simulink model "gs"  (Simulink 8.5)
settings: Solver=ode8  StartTime=0.0  StopTime=200  FixedStep=0.1  RelTol=1e-3
settings Model: Creator=Default  LastModifiedBy=Default
settings DataIOCC: SignalLoggingSaveFormat=Dataset
settings OptimizationCC: ExpressionDepthLimit=128
settings DebuggingCC: UnderspecifiedInitializationDetection=Simplified  MergeDetectMultiDrivingBlocksExec=error  FcnCallInpInsideContextMsg=EnableAllAsError  StateNameClashWarn=none
settings GRTTargetCC: CombineOutputUpdateFcns=on  GRTInterface=off

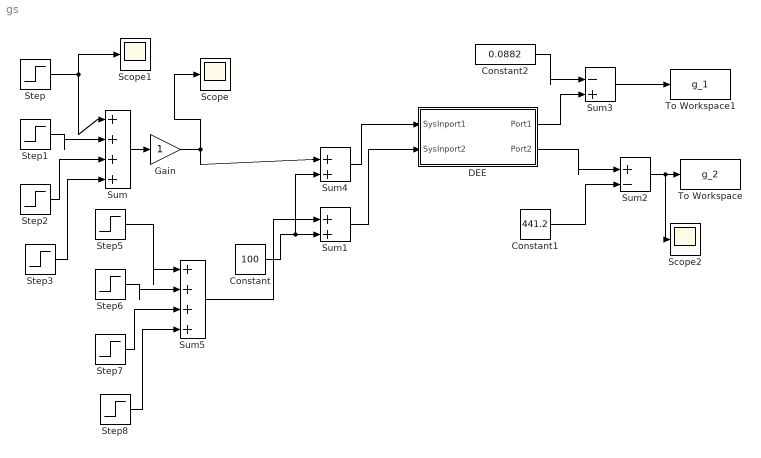
== system gs ==
  Constant : Constant  Value=100
  Constant1 : Constant  Value=441.2
  Constant2 : Constant  Value=0.0882
  DEE : Subsystem  mask(Differential Equation Editor (DEE)){}
      settings: OpenFcn=diffeqed
      mask Display: disp('Differential Equation\n Editor')
  Gain : Gain
  Scope : Scope
  Scope1 : Scope
  Scope2 : Scope
      settings: SaveName=ScopeData2
  Step : Step  Time=20  SampleTime=0
  Step1 : Step  Time=40  After=-1  SampleTime=0
  Step2 : Step  Time=60  After=-1  SampleTime=0
  Step3 : Step  Time=80  SampleTime=0
  Step5 : Step  Time=120  SampleTime=0
  Step6 : Step  Time=140  After=-1  SampleTime=0
  Step7 : Step  Time=160  After=-1  SampleTime=0
  Step8 : Step  Time=180  SampleTime=0
  Sum : Sum  Inputs=|++++
  Sum1 : Sum  Inputs=|++
  Sum2 : Sum  Inputs=|+-
  Sum3 : Sum  Inputs=|-+
  Sum4 : Sum  Inputs=|++
  Sum5 : Sum  Inputs=|++++
  To Workspace : ToWorkspace  VariableName=g_2  SampleTime=-1
  To Workspace1 : ToWorkspace  VariableName=g_1  SampleTime=-1
  wires:
  Step/1 -> Sum/1, Scope1/1
  Step1/1 -> Sum/2
  Step2/1 -> Sum/3
  Step3/1 -> Sum/4
  Sum/1 -> Gain/1
  Constant/1 -> Sum4/2, Sum1/2
  Constant1/1 -> Sum2/2
  Sum2/1 -> Scope2/1, To Workspace/1
  DEE/2(Port2) -> Sum2/1
  DEE/1(Port1) -> Sum3/2
  Constant2/1 -> Sum3/1
  Sum3/1 -> To Workspace1/1
  Gain/1 -> Scope/1, Sum4/1
  Sum4/1 -> DEE/1(SysInport1)
  Step5/1 -> Sum5/1
  Step6/1 -> Sum5/2
  Step7/1 -> Sum5/3
  Step8/1 -> Sum5/4
  Sum5/1 -> Sum1/1
  Sum1/1 -> DEE/2(SysInport2)

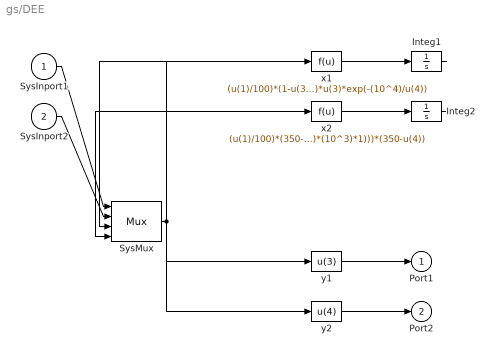
== system gs/DEE ==
  SysInport1 : Inport
  SysInport2 : Inport  Port=2
  Integ1 : Integrator  InitialCondition=0.0882
  Integ2 : Integrator  InitialCondition=441.2
  SysMux : Mux
  x1 : Fcn  Expr=(u(1)/100)*(1-u(3))-(7.2*10^10)*u(3)*exp(-(10^4)/u(4))
  x2 : Fcn  Expr=(u(1)/100)*(350-u(4))-((-(2*10^5)/(10^3))*(7.2*10^10)*u(3)*exp(-(10^4)/u(4)))+(((10^3)*1)/((10^3)*100))*(u(2))*(1-exp(-(7*10^5)/(u(2)*(10^3)*1)))*(350-u(4))
  y1 : Fcn  Expr=u(3)
  y2 : Fcn  Expr=u(4)
  Port1 : Outport
  Port2 : Outport  Port=2
  wires:
  SysInport1/1 -> SysMux/1
  SysInport2/1 -> SysMux/2
  SysMux/1 -> x1/1, x2/1, y1/1, y2/1
  x1/1 -> Integ1/1
  Integ1/1 -> SysMux/3
  x2/1 -> Integ2/1
  Integ2/1 -> SysMux/4
  y1/1 -> Port1/1
  y2/1 -> Port2/1
